simulink model "OLRF"  (R2023a)
settings: Solver=VariableStepAuto  StartTime=0.0  StopTime=10.0  RelTol=1e-3
values from neighbouring files (symbols this model uses):
  b = 0.490    (= 0.49)    [Cascaded_PI_Step.m]    (also in Cascaded_PI_Zero_Ref.m; Gain_Scheduled_PI_Step.m; Gain_Scheduled_PI_Zero_Ref.m; Inner_Loop_Relay_Feedback.m)
  Clda = 0.65    [Cascaded_PI_Step.m]    (also in Cascaded_PI_Zero_Ref.m; Gain_Scheduled_PI_Step.m; Gain_Scheduled_PI_Zero_Ref.m; Inner_Loop_Relay_Feedback.m)
  Clo = 1.108    [Cascaded_PI_Step.m]    (also in Cascaded_PI_Zero_Ref.m; Gain_Scheduled_PI_Step.m; Gain_Scheduled_PI_Zero_Ref.m; Inner_Loop_Relay_Feedback.m)
  Clp = -1.5    [Cascaded_PI_Step.m]    (also in Cascaded_PI_Zero_Ref.m = -11.5; Gain_Scheduled_PI_Step.m = -11.5; Gain_Scheduled_PI_Zero_Ref.m = -11.5; Inner_Loop_Relay_Feedback.m = -11.5)
  KT2 = 3    [Outer_Loop_Relay_Feedback.m]
  phi_des = 30    [Cascaded_PI_Step.m]    (also in Cascaded_PI_Zero_Ref.m = 0; Gain_Scheduled_PI_Step.m; Gain_Scheduled_PI_Zero_Ref.m = 0; Outer_Loop_Relay_Feedback.m = 20)
  rho = 1.204    [Cascaded_PI_Step.m]    (also in Cascaded_PI_Zero_Ref.m; Gain_Scheduled_PI_Step.m; Gain_Scheduled_PI_Zero_Ref.m; Inner_Loop_Relay_Feedback.m)
  S = 0.44    [Cascaded_PI_Step.m]    (also in Cascaded_PI_Zero_Ref.m; Gain_Scheduled_PI_Step.m; Gain_Scheduled_PI_Zero_Ref.m; Inner_Loop_Relay_Feedback.m)
  Va = 15    [Cascaded_PI_Step.m]    (also in Cascaded_PI_Zero_Ref.m; Gain_Scheduled_PI_Step.m; Gain_Scheduled_PI_Zero_Ref.m; Inner_Loop_Relay_Feedback.m)
libraries: slpidlib x1
settings Model: Creator=brend  LastModifiedBy=brend

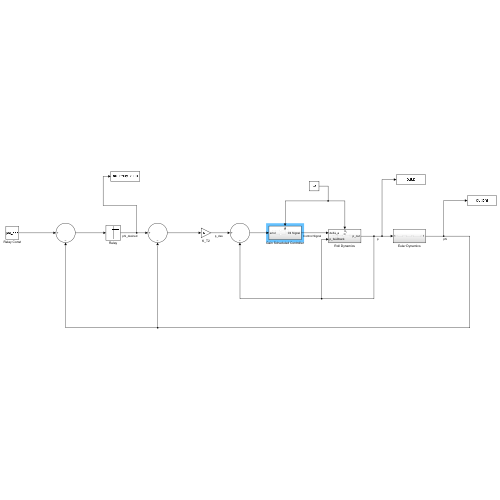
[thumbnail: Simulink's stored preview of the top-level diagram]
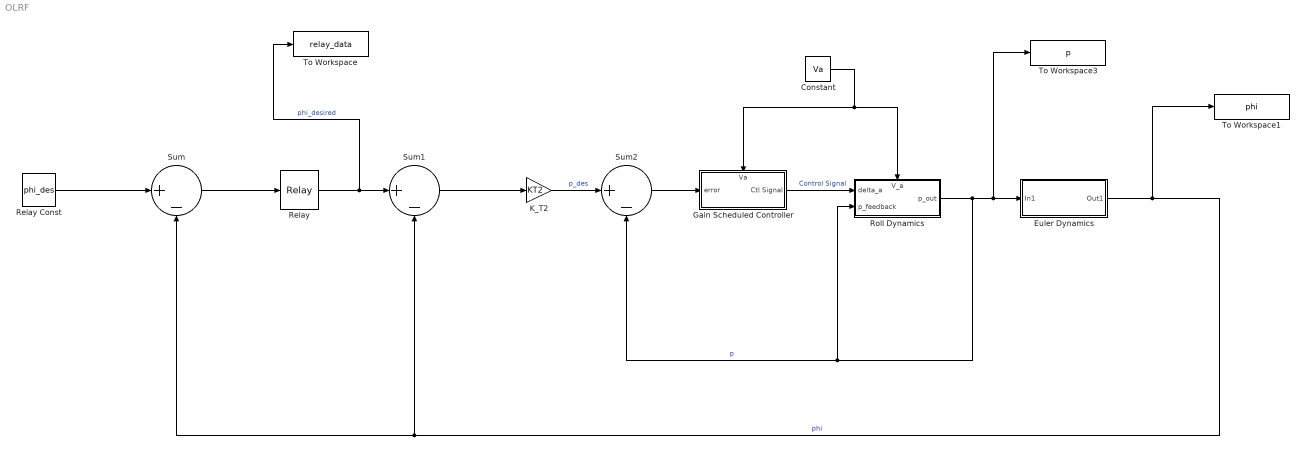
== system OLRF ==
  Constant : Constant  Value=Va
  Euler Dynamics : Subsystem
  Gain Scheduled Controller : Subsystem
      settings: PortSchema="{\"entries\":[{\"content\":{\"sides\":[{\"content\":{\"connectorIds\":[\"In1\"]},\"type\":\"ConnectorPlacement.EquallySpacedRectSide\",\"uuid\":\"2e087caa-f72d-4490-8964-36fbcf7716d7\"},{\"content\":{\"connectorIds\":[\"Out1\"],\"side\":\"RIGHT\"},\"type\":\"ConnectorPlacement.EquallySpacedRectSide\",\"uuid\":\"b0dafe2c-6d7a-42e1-bf72-883c5565d2ef\"},{\"content\":{\"connectorIds\":[\"In2\"],\"side\":\"TOP\"},\"type\":\"ConnectorPlacement.EquallySpacedRectSide\",\"uuid\":\"4416cd10-6726-4ba3-b71a-642a6449d506\"}]},\"type\":\"ConnectorPlacement.EquallySpacedConnector\",\"uuid\":\"4db1e7fb-938c-4dd4-ad91-0eb120ffb4c4\"}],\"packageUris\":[\"http://schema.mathworks.com/mf0/Connector/R2020b\"],\"version\":\"1.0\"}"
  K_T2 : Gain  Gain=KT2
  Relay : Relay  OnSwitchValue=30  OffSwitchValue=10  OnOutputValue=phi_des  OffOutputValue=-phi_des
  Relay Const : Constant  Value=phi_des
  Roll Dynamics : Subsystem
      settings: PortSchema="{\"entries\":[{\"content\":{\"sides\":[{\"content\":{\"connectorIds\":[\"In1\",\"In2\"]},\"type\":\"ConnectorPlacement.EquallySpacedRectSide\",\"uuid\":\"0ac85a74-38c1-4d65-b1c0-9ca36de2cddb\"},{\"content\":{\"connectorIds\":[\"Out1\"],\"side\":\"RIGHT\"},\"type\":\"ConnectorPlacement.EquallySpacedRectSide\",\"uuid\":\"84e324c4-b4ec-429b-b00b-3022433bb281\"},{\"content\":{\"connectorIds\":[\"In3\"],\"side\":\"TOP\"},\"type\":\"ConnectorPlacement.EquallySpacedRectSide\",\"uuid\":\"b4486eb0-6e0f-4f77-80f0-5dbcf5ffe993\"}]},\"type\":\"ConnectorPlacement.EquallySpacedConnector\",\"uuid\":\"7fd31f13-990e-44ec-9889-e700ea070706\"}],\"packageUris\":[\"http://schema.mathworks.com/mf0/Connector/R2020b\"],\"version\":\"1.0\"}"
  Sum : Sum  Inputs=|+-
  Sum1 : Sum  Inputs=|+-
  Sum2 : Sum  Inputs=|+-
  To Workspace : ToWorkspace  VariableName=relay_data  SaveFormat=Timeseries  SampleTime=-1
  To Workspace1 : ToWorkspace  VariableName=phi  SaveFormat=Timeseries  SampleTime=-1
  To Workspace3 : ToWorkspace  VariableName=p  SaveFormat=Timeseries  SampleTime=-1
  wires:
  Relay Const/1 -> Sum/1
  Sum/1 -> Relay/1
  Relay/1 -> Sum1/1, To Workspace/1  "phi_desired"
  Sum1/1 -> K_T2/1
  K_T2/1 -> Sum2/1  "p_des"
  Gain Scheduled Controller/1(Ctl Signal) -> Roll Dynamics/1(delta_a)  "Control Signal"
  Roll Dynamics/1(p_out) -> To Workspace3/1, Euler Dynamics/1(In1), Roll Dynamics/2(p_feedback), Sum2/2  "p"
  Sum2/1 -> Gain Scheduled Controller/1(error)
  Euler Dynamics/1(Out1) -> Sum1/2, Sum/2, To Workspace1/1  "phi"
  Constant/1 -> Gain Scheduled Controller/2(Va), Roll Dynamics/3(V_a)

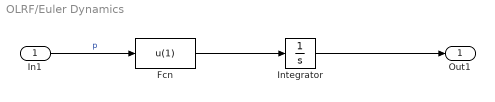
== system OLRF/Euler Dynamics ==
  In1 : Inport
  Fcn : Fcn  Expr=u(1)
  Integrator : Integrator
  Out1 : Outport
  wires:
  In1/1 -> Fcn/1  "p"
  Integrator/1 -> Out1/1
  Fcn/1 -> Integrator/1

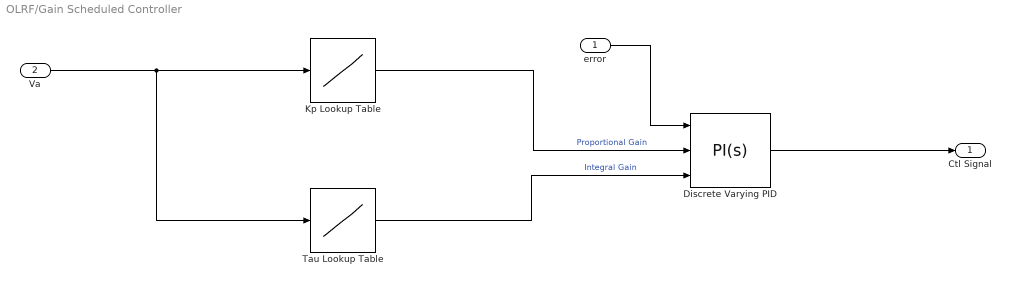
== system OLRF/Gain Scheduled Controller ==
  error : Inport
  Va : Inport  Port=2
  Discrete Varying PID : slpidlib/PID Controller  Controller=PI  Form=Parallel  TimeDomain=Continuous-time  UseExternalTs=off  SampleTime=-1  IntegratorMethod=Forward Euler  FilterMethod=Forward Euler  ControllerParametersSource=external  P=1  I=1  UseKiTs=off  D=0  N=100  UseFilter=on  TunerSelectOption=Transfer Function Based (PID Tuner App)  InitialConditionSource=internal  InitialConditionForIntegrator=0  InitialConditionForFilter=0  DifferentiatorICPrevScaledInput=0  ExternalReset=none  TrackingMode=off  Kt=1  LimitOutput=off  SatLimitsSource=internal  UpperSaturationLimit=inf  LowerSaturationLimit=-inf  LinearizeAsGain=on  AntiWindupMode=none  Kb=1  LimitIntegrator=off  UpperIntegratorSaturationLimit=inf  LowerIntegratorSaturationLimit=-inf  POutMin=[]  POutMax=[]  IOutMin=[]  IOutMax=[]  DOutMin=[]  DOutMax=[]  NOutMin=[]  NOutMax=[]  SumOutMin=[]  SumOutMax=[]  SaturationOutMin=[]  SaturationOutMax=[]  PParamMin=[]  PParamMax=[]  IParamMin=[]  IParamMax=[]  DParamMin=[]  DParamMax=[]  NParamMin=[]  NParamMax=[]  KbParamMin=[]  KbParamMax=[]  KtParamMin=[]  KtParamMax=[]  KbOutMin=[]  KbOutMax=[]  KtOutMin=[]  KtOutMax=[]  IntegratorOutMin=[]  IntegratorOutMax=[]  FilterOutMin=[]  FilterOutMax=[]  SumI1OutMin=[]  SumI1OutMax=[]  SumI2OutMin=[]  SumI2OutMax=[]  SumI3OutMin=[]  SumI3OutMax=[]  SumI4OutMin=[]  SumI4OutMax=[]  SumDOutMin=[]  SumDOutMax=[]  DifferentiatorOutMin=[]  DifferentiatorOutMax=[]  FilterDiffOutCoefMin=[]  FilterDiffOutCoefMax=[]  ReciprocalOutMin=[]  ReciprocalOutMax=[]  SumDenOutMin=[]  SumDenOutMax=[]  SumNumOutMin=[]  SumNumOutMax=[]  DivideOutMin=[]  DivideOutMax=[]  UdiffTsProdOutMin=[]  UdiffTsProdOutMax=[]  NTsProdOutMin=[]  NTsProdOutMax=[]  UintegralTsProdOutMin=[]  UintegralTsProdOutMax=[]  UngainTsProdOutMin=[]  UngainTsProdOutMax=[]  ClampingZeroOutDataTypeStr=Inherit: Inherit via back propagation  ClampingZeroOutMin=[]  ClampingZeroOutMax=[]  FilterDenConstantOutDataTypeStr=Inherit: Inherit via back propagation  FilterDenConstantOutMin=[]  FilterDenConstantOutMax=[]  PCopyOutDataTypeStr=Inherit: Inherit via back propagation  PCopyOutMin=[]  PCopyOutMax=[]  NCopyOutDataTypeStr=Inherit: Inherit via back propagation  NCopyOutMin=[]  NCopyOutMax=[]  IntegratorContinuousStateAttributes=''  IntegratorStateMustResolveToSignalObject=off  IntegratorRTWStateStorageClass=Auto  FilterContinuousStateAttributes=''  FilterStateMustResolveToSignalObject=off  FilterRTWStateStorageClass=Auto  ParallelPVariant=ExternalParameters  IdealPVariant=Disabled  IVariant=ExternalParameters  DVariant=Disabled  IntegratorVariant=Continuous  SatVariant=Disabled  AWVariant=Passthrough  PCopyVariant=Disabled  TRVariant=Disabled  FdbkBlocksVariant=Forward  IdealPFdbkVariant=Disabled  SatFdbkVariant=Disabled  DerivativeFilterVariant=Disabled  NVariant=Disabled  NCopyVariant=Disabled_SignalSpec  FilterICVariant=Disabled  IntegratorICVariant=InternalICs  ExternalResetVariant=Disabled  TRSumVariant=Passthrough  SumFdbkVariant=Disabled  SumVariant=Sum_PI  TsampFilterVariant=InternalTs  TsampNgainVariant=Passthrough  TsampIntegralVariant=Disabled_SignalSpec  ExternalSaturationOutDataTypeStr=Inherit: Same as second input
      settings: LibrarySourceBlock=cstblocks/Linear Parameter Varying/Discrete Varying PID
  Kp Lookup Table : Lookup_n-D  NumberOfTableDimensions=1  BreakpointsForDimension1=[7,10,15]  Table=[0.92, 0.23, 0.16]  InternalRulePriority=Speed  RndMeth=Simplest
  Tau Lookup Table : Lookup_n-D  NumberOfTableDimensions=1  BreakpointsForDimension1=[7,10,15]  Table=[0.095,0.146,0.178]  InternalRulePriority=Speed  RndMeth=Simplest
  Ctl Signal : Outport
  wires:
  Va/1 -> Tau Lookup Table/1, Kp Lookup Table/1
  Kp Lookup Table/1 -> Discrete Varying PID/2  "Proportional Gain"
  Tau Lookup Table/1 -> Discrete Varying PID/3  "Integral Gain"
  error/1 -> Discrete Varying PID/1
  Discrete Varying PID/1 -> Ctl Signal/1

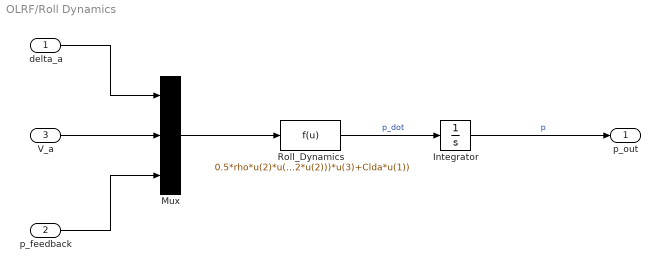
== system OLRF/Roll Dynamics ==
  delta_a : Inport
  p_feedback : Inport  Port=2
  V_a : Inport  Port=3
  Integrator : Integrator
  Mux : Mux  Inputs=3
  Roll_Dynamics : Fcn  Expr=0.5*rho*u(2)*u(2)*S*b*(Clo + Clp*(b/(2*u(2)))*u(3)+Clda*u(1))
  p_out : Outport
  wires:
  delta_a/1 -> Mux/1
  Mux/1 -> Roll_Dynamics/1
  Integrator/1 -> p_out/1  "p"
  V_a/1 -> Mux/2
  p_feedback/1 -> Mux/3
  Roll_Dynamics/1 -> Integrator/1  "p_dot"
